simulink model "PSD_linecodes_2020a"  (R2020b)
settings: Solver=VariableStepDiscrete  StartTime=0.0  StopTime=20000  RelTol=1e-3  EnableMultiTasking=on
PreLoadFcn:
  | T=1;
  | Ts=T/8;
libraries: dspobslib x3, dspstat3 x3, commutil2 x1, commrandsrc2 x1
settings Model: Creator=morelos_zaragoza  LastModifiedBy=14083
settings DataIOCC: LimitDataPoints=on  SaveFormat=Array  SignalLoggingSaveFormat=ModelDataLogs  ReturnWorkspaceOutputs=off
settings OptimizationCC: ExpressionDepthLimit=2147483647  InitFltsAndDblsToZero=on  LifeSpan=inf
settings DebuggingCC: SaveWithParameterizedLinksMsg=none  UnderspecifiedInitializationDetection=Classic  MergeDetectMultiDrivingBlocksExec=none  SignalResolutionControl=TryResolveAllWithWarning  SolverPrmCheckMsg=warning  MultiTaskDSMMsg=warning  MultiTaskCondExecSysMsg=none  FcnCallInpInsideContextMsg=warning  StateNameClashWarn=warning  SFUnexpectedBacktrackingDiag=warning  SFNoUnconditionalDefaultTransitionDiag=warning  SFExecutionAtInitializationDiag=none  ArithmeticOperatorsInVariantConditions=warning
settings HardwareCC: ProdBitPerPointer=32  ProdBitPerSizeT=32  ProdBitPerPtrDiffT=32  ProdLargestAtomicFloat=None  ProdIntDivRoundTo=Undefined  ProdEndianess=Unspecified  ProdWordSize=32  ProdHWDeviceType=32-bit Generic
settings ModelReferenceCC: PropagateSignalLabelsOutOfModel=off
settings SFSimCC: SimUseLocalCustomCode=off  CustomCodeUndefinedFunction=UseInterfaceOnly
settings RTWCC: RTWUseLocalCustomCode=off
settings CodeAppCC: StateflowObjectComments=on
settings GRTTargetCC: TargetFcnLib=ansi_tfl_tmw.mat  TargetLangStandard=C89/C90 (ANSI)  CombineOutputUpdateFcns=off  GRTInterface=on
settings ConfigComp: CovMetricSettings=dw  CovSaveCumulativeToWorkspaceVar=on  CovSaveSingleToWorkspaceVar=on  CovExternalEMLEnable=off

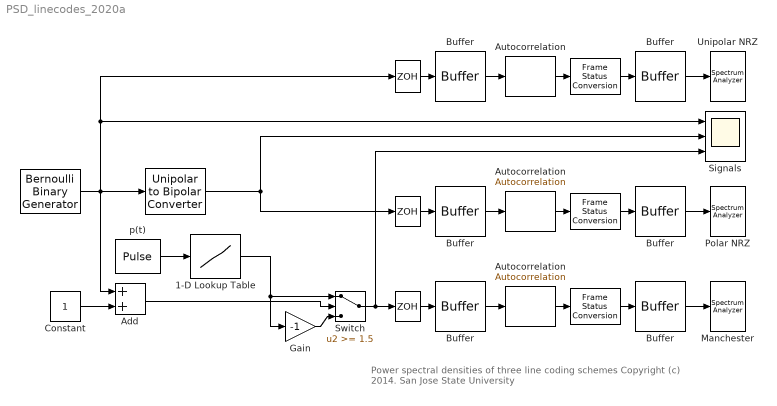
== system PSD_linecodes_2020a ==
  note: Power spectral densities of three line coding schemes
      | Copyright (c) 2014. San Jose State University
  " " : ZeroOrderHold  SampleTime=Ts
  "   " : commutil2/Unipolar to Bipolar Converter  M=2  polarity=Positive  dataType=Inherit via internal rule
  " " : ZeroOrderHold  SampleTime=Ts
  "    " : commrandsrc2/Bernoulli Binary Generator  P=0.5  seed=61173111  Ts=T  frameBased=off  sampPerFrame=1  orient=off  outDataType=double
      settings: SourceProductBaseCode=CM
  "       " : dspobslib/Frame Status Conversion  growRefPort=off  outframe=Frame-based
      settings: SourceProductBaseCode=DS
  "         " : dspobslib/Frame Status Conversion  growRefPort=off  outframe=Frame-based
      settings: SourceProductBaseCode=DS
  " " : ZeroOrderHold  SampleTime=Ts
  "               " : dspobslib/Frame Status Conversion  growRefPort=off  outframe=Frame-based
      settings: SourceProductBaseCode=DS
  "      Buffer      " : Buffer  N=1
  "     Buffer     " : Buffer  N=1024
  "    Buffer    " : Buffer  N=1
  "   Buffer   " : Buffer  N=1024
  "  Autocorrelation  " : dspstat3/Autocorrelation  AllPositiveLags=on  maxlag=1  bias=None  domain=Time  roundingMode=Floor  overflowMode=off  outputDataTypeStr=Inherit: Same as accumulator  outputMin=[]  outputMax=[]  outputLastDataTypeStr=Inherit: Same as accumulator
      settings: SourceProductBaseCode=DS
  "  Buffer  " : Buffer  N=1
  " Autocorrelation " : dspstat3/Autocorrelation  AllPositiveLags=on  maxlag=1  bias=None  domain=Time  roundingMode=Floor  overflowMode=off  outputDataTypeStr=Inherit: Same as accumulator  outputMin=[]  outputMax=[]  outputLastDataTypeStr=Inherit: Same as accumulator
      settings: SourceProductBaseCode=DS
  " Buffer " : Buffer  N=1024
  1-D Lookup Table : Lookup_n-D  NumberOfTableDimensions=1  BreakpointsForDimension1=[0,1]  Table=[-1,1]  RndMeth=Simplest  InputSameDT=on
  Add : Sum
  Autocorrelation : dspstat3/Autocorrelation  AllPositiveLags=on  maxlag=1  bias=None  domain=Time  roundingMode=Floor  overflowMode=off  outputDataTypeStr=Inherit: Same as accumulator  outputMin=[]  outputMax=[]  outputLastDataTypeStr=Inherit: Same as accumulator
      settings: SourceProductBaseCode=DS
  Constant : Constant
  Gain : Gain  Gain=-1
  Manchester : SpectrumAnalyzer
  Polar NRZ : SpectrumAnalyzer
  Signals : Scope  NumInputPorts=3
  Switch : Switch  Threshold=1.5
  Unipolar NRZ : SpectrumAnalyzer
  p(t) : DiscretePulseGenerator  PulseType=Time based  Period=T  PulseWidth=50
  wires:
  "    "/1 -> "   "/1, Signals/1, " "/1, Add/1
  "   "/1 -> " "/1, Signals/2
  Autocorrelation/1 -> "       "/1
  " Buffer "/1 -> Autocorrelation/1
  "   Buffer   "/1 -> " Autocorrelation "/1
  "  Buffer  "/1 -> Unipolar NRZ/1
  "       "/1 -> "  Buffer  "/1
  "         "/1 -> "    Buffer    "/1
  " Autocorrelation "/1 -> "         "/1
  "    Buffer    "/1 -> Polar NRZ/1
  " "/1 -> " Buffer "/1
  " "/1 -> "   Buffer   "/1
  p(t)/1 -> 1-D Lookup Table/1
  Constant/1 -> Add/2
  Add/1 -> Switch/2
  Switch/1 -> Signals/3, " "/1
  Gain/1 -> Switch/3
  "     Buffer     "/1 -> "  Autocorrelation  "/1
  "               "/1 -> "      Buffer      "/1
  "  Autocorrelation  "/1 -> "               "/1
  "      Buffer      "/1 -> Manchester/1
  " "/1 -> "     Buffer     "/1
  1-D Lookup Table/1 -> Gain/1, Switch/1
